simulink model "Pendulum"  (Simulink 7.0)
settings: Solver=ode1  StartTime=0.0  StopTime=inf  FixedStep=0.01  RelTol=1e-3
undefined symbols (not defined in the file or in its folder): plot_pend
libraries: mblibv1 x9, quarc_library x1
settings Model: Creator=colinlea  LastModifiedBy=colinlea  ExtModeTrigDuration=10000
settings SolverCC: PositivePriorityOrder=on
settings RTWCC: SystemTargetFile=quarc_windows.tlc  TemplateMakefile=quarc_default_tmf  Description=QuaRC Win32 Target  ProcessScript=quarc_windows_make_rtw_hook
settings STFCustomTargetCC: TargetPreCompLibLocation=C:\DOCUME~1\ALLUSE~1\APPLIC~1\QuaRC\lib\2007b\windows\release  GenFloatMathFcnCalls=ANSI_C  SystemTargetFile=quarc_windows.tlc
settings GRTTargetCC: TargetPreCompLibLocation=C:\DOCUME~1\ALLUSE~1\APPLIC~1\QuaRC\lib\2007b\windows\release  CompOptLevelCompliant=off  MatFileLogging=off  ExtMode=on  ExtModeMexFile=quarc_comm

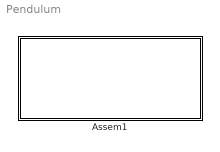
== system Pendulum ==
  Assem1 : Subsystem

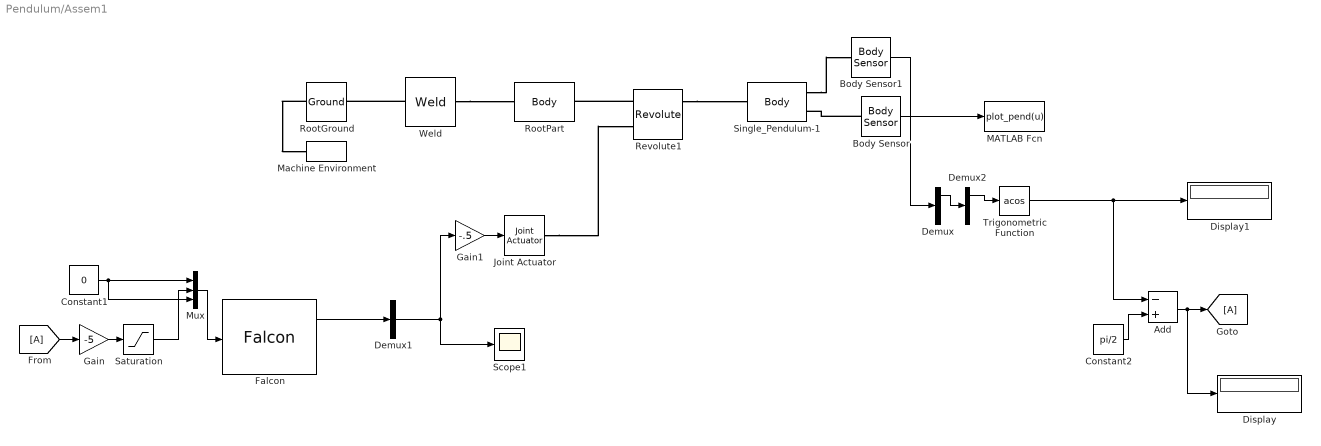
== system Pendulum/Assem1 ==
  Add : Sum  Inputs=-+  OutDataType=sfix(16)  OutScaling=2^-10
  Body Sensor : mblibv1/Sensors &  Actuators/Body Sensor  DialogController=MECH.DynMechDlgSource  SystemSampleTime=-1  PhysicalDomain=Mechanical  PortType=blob  Muxed=on  Pose=off  Angle=on  AngleUnits=deg  ArcVelocity=off  ArcVelocityUnits=deg/s  ArcAcceleration=off  ArcAccelerationUnits=deg/s^2  CoordPosition=on  CoordPositionUnits=cm  Velocity=off  VelocityUnits=m/s  Acceleration=off  AccelerationUnits=m/s^2  Quaternion=on  QuaternionDT=off  QuaternionDDT=off  QuaternionUnits=off  OutputVector=[1]  ActiveIO=on  Width=3  DialogClass=MechanicalSensorBlock  ReferenceFrame=Absolute (World)
  Body Sensor1 : mblibv1/Sensors &  Actuators/Body Sensor  DialogController=MECH.DynMechDlgSource  SystemSampleTime=-1  PhysicalDomain=Mechanical  PortType=blob  Muxed=on  Pose=on  Angle=on  AngleUnits=deg  ArcVelocity=off  ArcVelocityUnits=deg/s  ArcAcceleration=off  ArcAccelerationUnits=deg/s^2  CoordPosition=off  CoordPositionUnits=m  Velocity=off  VelocityUnits=m/s  Acceleration=off  AccelerationUnits=m/s^2  Quaternion=on  QuaternionDT=off  QuaternionDDT=off  QuaternionUnits=off  OutputVector=[1]  ActiveIO=on  Width=9  DialogClass=MechanicalSensorBlock  ReferenceFrame=Absolute (World)
  Constant1 : Constant  Value=0  OutDataType=sfix(16)  OutScaling=2^0
  Constant2 : Constant  Value=pi/2  OutDataType=sfix(16)  OutScaling=2^0
  Demux : Demux  Outputs=3
  Demux1 : Demux  Outputs=3
  Demux2 : Demux  Outputs=3
  Display : Display
  Display1 : Display
  Falcon : quarc_library/Devices/Third-Party/Novint/Falcon  sample_time=qc_get_step_size  show_calibrate=off
  Gain : Gain  Gain=-5  ParameterDataType=sfix(16)  ParameterScaling=2^0  OutDataType=sfix(16)  OutScaling=2^0
  Gain1 : Gain  Gain=-.5  ParameterDataType=sfix(16)  ParameterScaling=2^0  OutDataType=sfix(16)  OutScaling=2^0
  Joint Actuator : mblibv1/Sensors &  Actuators/Joint Actuator  DialogController=MECH.DynMechDlgSource  SystemSampleTime=-1  PhysicalDomain=Mechanical  PortType=blob  ActuationStyle=Force  AngleUnits=deg  ArcVelocityUnits=deg/s  ArcAccelerationUnits=deg/s^2  CoordPositionUnits=m  VelocityUnits=m/s  AccelerationUnits=m/s^2  ForceUnits=N  TorqueUnits=N*m  ActiveIO=on  Width=1  DialogClass=MechanicalActuatorBlock  Primitive=R1  ReferenceFrame=Absolute (World)
  MATLAB Fcn : MATLABFcn  MATLABFcn=plot_pend(u)  OutputDimensions=0  OutputSignalType=real
  Machine Environment : mblibv1/Bodies/Machine Environment  Orientation=left  DialogController=MECH.DialogSource  SystemSampleTime=-1  PortType=env  PhysicalDomain=Mechanical  DialogTemplateClass=MECH.MachineEnvironment  SyncWhenCopied=off  Gravity=[0 -9.81 0]  GravityUnits=m/s^2  GravityAsSignal=off  Dimensionality=Auto-detect  AnalysisType=Forward dynamics  LinearAssemblyTolerance=1e-3  LinearAssemblyToleranceUnits=m  AngularAssemblyTolerance=1e-3  AngularAssemblyToleranceUnits=rad  ConstraintSolverType=Stabilizing  ConstraintRelTolerance=1e-4  ConstraintAbsTolerance=1e-4  UseRobustSingularityHandling=off  RedundancyAnalysisToleranceType=Automatically select tolerance  RedundancyAnalysisTolerance=1e-14  StatePerturbationType=Fixed  PerturbationSize=1e-5  VisualizeMachine=on
  Mux : Mux  Inputs=3
  Revolute1 : mblibv1/Joints/Revolute  DialogController=MECH.DynMechDlgSource  PhysicalDomain=mechanical  SubClassName=Unknown  LeftPortType=blob  RightPortType=blob  LConnTagsString=__newl0|SA1  RConnTagsString=__newr0|SA1  NumSAPorts=2  CutJoint=off  MarkAsCut=off  Primitives=prismatic  PrimitiveProps=R1$World$[0 0 1]$revolute  DialogClass=JointBlock  R1Axis=[0 0 1]
  RootGround : mblibv1/Bodies/Ground  DialogController=MECH.DynMechDlgSource  SystemSampleTime=-1  LeftPortType=env  RightPortType=workingframe  PhysicalDomain=Mechanical  DialogClass=GroundBlock  CoordPosition=[0.00021789 0.0021105 -0.0062052]  CoordPositionUnits=m  StateVectorMgrId=-1  MachineId=[0 0]  ShowEnvPort=on
  RootPart : mblibv1/Bodies/Body  DialogController=MECH.DynMechDlgSource  PhysicalDomain=mechanical  SubClassName=Unknown  LeftPortType=workingframe  RightPortType=workingframe  LConnTagsString=CS3  RConnTagsString=CS2  DialogClass=MechanicalBodyBlock  Mass=0  MassUnits=kg  InertiaUnits=kg*m^2  Inertia=[0 0 0;0 0 0;0 0 0]  Shape=Cylinder  ShapeDims=[1 1]  ShapeUnits=m  ShapeUse=false  Density=1  DensityUnits=kg/m^3  DensityUse=false  CG=Right$CG$[0.00021789 0.0021105 -0.0062052]$WORLD$WORLD$m$[1 0 0;0 1 0;0 0 1]$3x3 Transform$rad$WORLD$false  WorkingFrames=Right$CS2$[0.00021789 0.0021105 -0.0062052]$WORLD$WORLD$m$[1 0 0;0 1 0;0 0 1]$3x3 Transform$rad$WORLD$true#Left$CS3$[0.00021789 0.0021105 -0.0062052]$WORLD$WORLD$m$[1 0 0;0 1 0;0 0 1]$3x3 Transform$rad$WORLD$true#Right$CS1$[0 0 0]$WORLD$WORLD$m$[1 0 0;0 1 0;0 0 1]$3x3 Transform$rad$WORLD$false  CGPos=[0.00021789 0.0021105 -0.0062052]  CGRot=[1 0 0;0 1 0;0 0 1]  CS0Pos=[]  CS0Rot=[]  CS1Pos=[0 0 0]  CS1Rot=[1 0 0;0 1 0;0 0 1]  CS2Pos=[0.00021789 0.0021105 -0.0062052]  CS2Rot=[1 0 0;0 1 0;0 0 1]  CS3Pos=[0.00021789 0.0021105 -0.0062052]  CS3Rot=[1 0 0;0 1 0;0 0 1]  CS4Pos=[]  CS4Rot=[]  CS5Pos=[]  CS5Rot=[]  CS6Pos=[]  CS6Rot=[]  CS7Pos=[]  CS7Rot=[]  CS8Pos=[]  CS8Rot=[]  CS9Pos=[]  CS9Rot=[]  CS10Pos=[]  CS10Rot=[]  CS11Pos=[]  CS11Rot=[]  CS12Pos=[]  CS12Rot=[]  CS13Pos=[]  CS13Rot=[]  CS14Pos=[]  CS14Rot=[]  CS15Pos=[]  CS15Rot=[]  CS16Pos=[]  CS16Rot=[]  CS17Pos=[]  CS17Rot=[]  CS18Pos=[]  CS18Rot=[]  CS19Pos=[]  CS19Rot=[]  CS20Pos=[]  CS20Rot=[]
  Saturation : Saturate  UpperLimit=4  LowerLimit=-4  OutDataType=sfix(16)  OutScaling=2^0
  Scope1 : Scope
      settings: TimeRange=10  YMin=-0.06  YMax=0.07
  Single_Pendulum-1 : mblibv1/Bodies/Body  DialogController=MECH.DynMechDlgSource  PhysicalDomain=mechanical  SubClassName=Unknown  LeftPortType=workingframe  RightPortType=workingframe  LConnTagsString=CS2  RConnTagsString=CS3|CS1  DialogClass=MechanicalBodyBlock  Mass=2  MassUnits=kg  InertiaUnits=kg*m^2  Inertia=[5.2218e-006 0 0;0 0.00024777 0;0 0 0.00024783]  Shape=Cylinder  ShapeDims=[1 1]  ShapeUnits=m  ShapeUse=false  Density=1  DensityUnits=kg/m^3  DensityUse=false  CG=Right$CG$[0.00021789 0.0021105 -0.0062052]$WORLD$WORLD$m$[1 0 0;0 1 0;0 0 1]$3x3 Transform$rad$WORLD$false  WorkingFrames=Right$CS3$[0.00021789 0.0021105 -0.0062052]$WORLD$WORLD$m$[1 0 0;0 1 0;0 0 1]$3x3 Transform$deg$WORLD$true#Left$CS2$[0.00021789 0.0021105 -0.0062052]$WORLD$WORLD$m$[1 0 0;0 1 0;0 0 1]$3x3 Transform$rad$WORLD$true#Right$CS1$[-0.033659 -0.0078895 0.023121]$WORLD$WORLD$m$[1 0 0;0 1 0;0 0 1]$3x3 Transform$rad$WORLD$true  CGPos=[0.00021789 0.0021105 -0.0062052]  CGRot=[1 0 0;0 1 0;0 0 1]  CS0Pos=[]  CS0Rot=[]  CS1Pos=[-0.033659 -0.0078895 0.023121]  CS1Rot=[1 0 0;0 1 0;0 0 1]  CS2Pos=[0.00021789 0.0021105 -0.0062052]  CS2Rot=[1 0 0;0 1 0;0 0 1]  CS3Pos=[0.00021789 0.0021105 -0.0062052]  CS3Rot=[1 0 0;0 1 0;0 0 1]  CS4Pos=[]  CS4Rot=[]  CS5Pos=[]  CS5Rot=[]  CS6Pos=[]  CS6Rot=[]  CS7Pos=[]  CS7Rot=[]  CS8Pos=[]  CS8Rot=[]  CS9Pos=[]  CS9Rot=[]  CS10Pos=[]  CS10Rot=[]  CS11Pos=[]  CS11Rot=[]  CS12Pos=[]  CS12Rot=[]  CS13Pos=[]  CS13Rot=[]  CS14Pos=[]  CS14Rot=[]  CS15Pos=[]  CS15Rot=[]  CS16Pos=[]  CS16Rot=[]  CS17Pos=[]  CS17Rot=[]  CS18Pos=[]  CS18Rot=[]  CS19Pos=[]  CS19Rot=[]  CS20Pos=[]  CS20Rot=[]
  Trigonometric Function : Trigonometry  Operator=acos
  Weld : mblibv1/Joints/Weld  DialogController=MECH.DynMechDlgSource  PhysicalDomain=mechanical  SubClassName=Unknown  LeftPortType=blob  RightPortType=blob  LConnTagsString=__newl0  RConnTagsString=__newr0  NumSAPorts=0  CutJoint=off  MarkAsCut=off  Primitives=weld  PrimitiveProps=W$WORLD$[0 0 0]$weld  DialogClass=JointBlock  WAxis=[0 0 0]
  wires:
  [A] -> Gain/1
  Falcon/1 -> Demux1/1
  Gain/1 -> Saturation/1
  Mux/1 -> Falcon/1
  Constant1/1 -> Mux/1, Mux/3
  Saturation/1 -> Mux/2
  Demux1/2 -> Scope1/1, Gain1/1
  Gain1/1 -> Joint Actuator/1
  Constant2/1 -> Add/2
  Add/1 -> [A], Display/1
  Body Sensor/1 -> MATLAB Fcn/1
  Body Sensor1/1 -> Demux/1
  Demux/1 -> Demux2/1
  Demux2/1 -> Trigonometric Function/1
  Trigonometric Function/1 -> Display1/1, Add/1
  connections:
  Revolute1/LConn1 -- RootPart/RConn1
  Weld/LConn1 -- RootGround/RConn1
  Weld/RConn1 -- RootPart/LConn1
  RootGround/LConn1 -- Machine Environment/RConn1
  Joint Actuator/RConn1 -- Revolute1/LConn2
  Body Sensor/LConn1 -- Single_Pendulum-1/RConn2
  Revolute1/RConn1 -- Single_Pendulum-1/LConn1
  Single_Pendulum-1/RConn1 -- Body Sensor1/LConn1
